simulink model "batModel"  (R2022a)
settings: Solver=VariableStepAuto  StartTime=0.0  StopTime=10.0  RelTol=1e-3
settings Model: Creator=JadKHaddad  LastModifiedBy=JadKHaddad

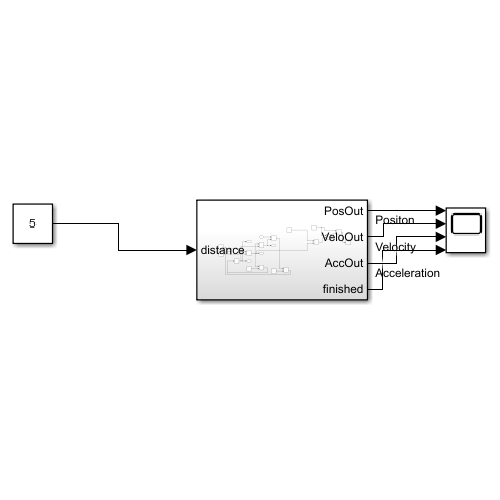
[thumbnail: Simulink's stored preview of the top-level diagram]
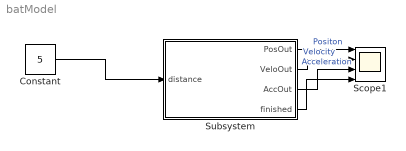
== system batModel ==
  Constant : Constant  Value=5
  Scope1 : Scope  NumInputPorts=4
  Subsystem : Subsystem
  wires:
  Subsystem/4(finished) -> Scope1/4
  Subsystem/3(AccOut) -> Scope1/3  "Acceleration"
  Subsystem/1(PosOut) -> Scope1/1  "Positon"
  Subsystem/2(VeloOut) -> Scope1/2  "Velocity"
  Constant/1 -> Subsystem/1(distance)

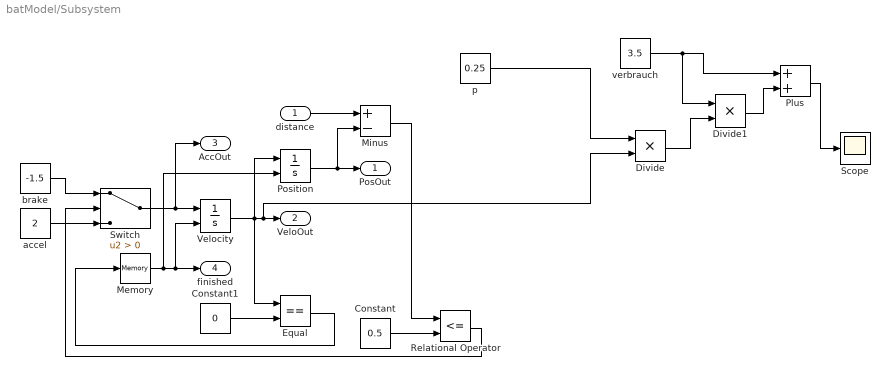
== system batModel/Subsystem ==
  distance : Inport
  Constant : Constant  Value=0.5
  Constant1 : Constant  Value=0
  Divide : Product  Inputs=**  RndMeth=Round
  Divide1 : Product  Inputs=**
  Equal : RelationalOperator  Operator===  OutDataTypeStr=boolean  RndMeth=Simplest  InputSameDT=off
  Memory : Memory
  Minus : Sum  Inputs=+-
  Plus : Sum
  Position : Integrator  ExternalReset=rising
  Relational Operator : RelationalOperator  Operator=<=  OutDataTypeStr=boolean  RndMeth=Simplest  InputSameDT=off
  Scope : Scope
  Switch : Switch  Criteria=u2 > Threshold  SaturateOnIntegerOverflow=off  InputSameDT=off
  Velocity : Integrator  ExternalReset=rising  LimitOutput=on  UpperSaturationLimit=1  LowerSaturationLimit=0
  accel : Constant  Value=2
  brake : Constant  Value=-1.5
  p : Constant  Value=0.25
  verbrauch : Constant  Value=3.5
  PosOut : Outport
  VeloOut : Outport  Port=2
  AccOut : Outport  Port=3
  finished : Outport  Port=4
  wires:
  Relational Operator/1 -> Switch/2
  brake/1 -> Switch/1
  Equal/1 -> Memory/1
  accel/1 -> Switch/3
  distance/1 -> Minus/1
  Minus/1 -> Relational Operator/1
  Constant1/1 -> Equal/2
  Constant/1 -> Relational Operator/2
  Memory/1 -> Velocity/2, finished/1, Position/2
  Position/1 -> Minus/2, PosOut/1
  Velocity/1 -> Divide/2, VeloOut/1, Equal/1, Position/1
  Switch/1 -> Velocity/1, AccOut/1
  p/1 -> Divide/1
  verbrauch/1 -> Divide1/1, Plus/1
  Divide/1 -> Divide1/2
  Divide1/1 -> Plus/2
  Plus/1 -> Scope/1
